simulink model "eleco2024"  (R2023a)
settings: Solver=VariableStepAuto  StartTime=0.0  StopTime=10.0  RelTol=1e-3
undefined symbols (not defined in the file or in its folder): Kd, Ki, Kp
libraries: checkpacklib x2, fod x1
settings Model: Creator=Hakan  LastModifiedBy=Hakan

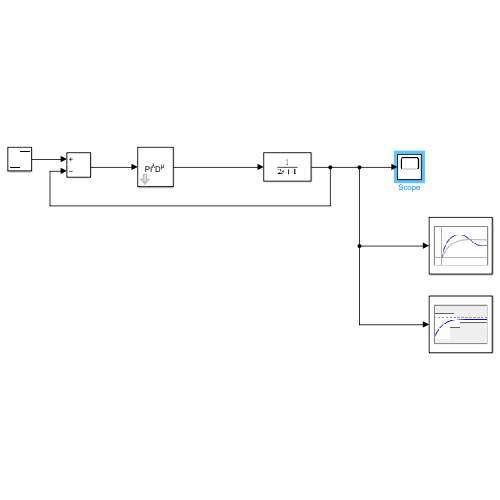
[thumbnail: Simulink's stored preview of the top-level diagram]
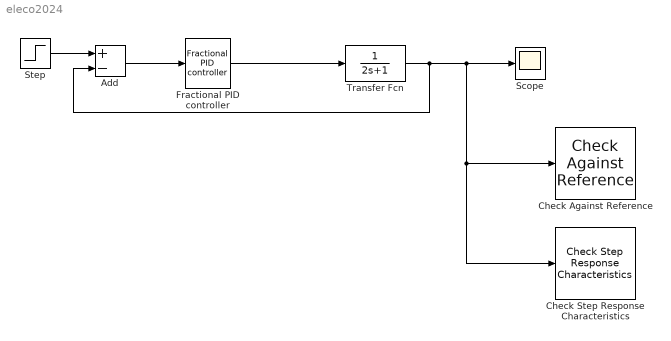
== system eleco2024 ==
  Add : Sum  Inputs=+-
  Check Against Reference : checkpacklib/Check Against Reference  InstantiateOnLoad=on  enabled=on  stopWhenAssertionFail=off  export=off  ViewDlgPos=[]  OpenViewOnLoad=off  LaunchViewOnOpen=off  TimeUnits=seconds  EnableReferenceBound=on  AbsTolerance=eps^(1/3)  RelTolerance=0.01  ReferenceTimes=linspace(0,10)  ReferenceAmplitudes=1-exp(-linspace(0,10)/2)
      settings: LibrarySourceBlock=sdolib/Model Verification/Check Against Reference
  Check Step Response Characteristics : checkpacklib/Check Step Response  Characteristics  InstantiateOnLoad=on  enabled=on  stopWhenAssertionFail=off  export=off  ViewDlgPos=[]  OpenViewOnLoad=off  LaunchViewOnOpen=off  TimeUnits=seconds  EnableStepResponseBound=on  InitialValue=0  FinalValue=1  StepTime=0  RiseTime=0.005  PercentRise=80  SettlingTime=0.007  PercentSettling=1  PercentOvershoot=1  PercentUndershoot=1
      settings: LibrarySourceBlock=|
      | sdolib/Model Verification/Check Step Response
      | Characteristics
  Fractional PID controller : fod/Fractional PID controller  Kp=Kp  Ki=Ki  lambda=lambda  Kd=Kd  mic=mu  freqRange=[0.001, 1000]  N=5
      settings: SourceProductName=FOMCON Toolbox
  Scope : Scope
  Step : Step  Before=1  SampleTime=0
  Transfer Fcn : TransferFcn  Denominator=[2 1]
  wires:
  Step/1 -> Add/1
  Add/1 -> Fractional PID controller/1
  Transfer Fcn/1 -> Check Step Response Characteristics/1, Check Against Reference/1, Scope/1, Add/2
  Fractional PID controller/1 -> Transfer Fcn/1
